simulink model "wiper_mil"  (R2018a)
settings: Solver=FixedStepDiscrete  StartTime=0.0  StopTime=10.0  FixedStep=1  RelTol=1e-3
undefined symbols (not defined in the file): sigbuilder_block
settings Model: Creator=Admin  LastModifiedBy=Admin
settings ConfigComp: CovEnable=on  RecordCoverage=on  CovMetricSettings=dcmwe  CovModelRefEnable=on

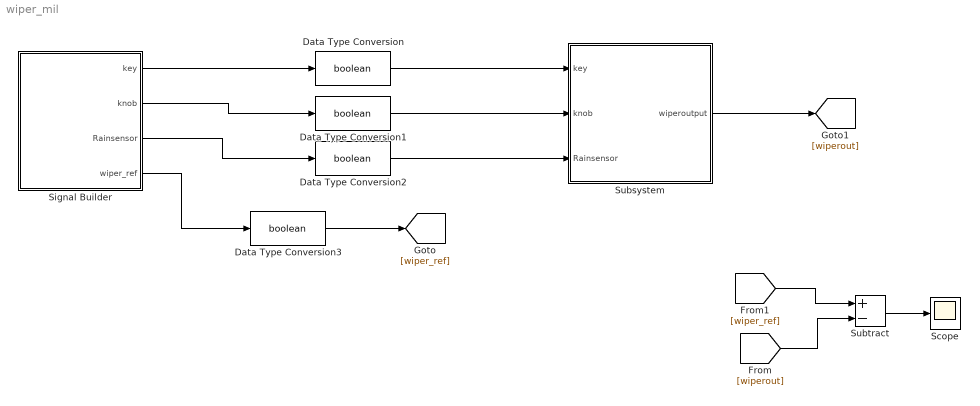
== system wiper_mil ==
  Data Type Conversion{,1..3} (4 alike) : DataTypeConversion  OutDataTypeStr=boolean
  Scope : Scope
  Signal Builder : Subsystem  Tag=STV Subsys  LoadFcn=sigbuilder_block('load',[440.25 156.75 544.5 355.5 ]);  StartFcn=sigbuilder_block('start');  StopFcn=sigbuilder_block('stop');  ClipboardFcn=sigbuilder_block('clipboard');  mask(Sigbuilder block){tuvar=[0:10]}
      mask help: Simulink:masks:SigbuilderBlock_MD
      mask init:
      | if ~strcmp(get_param(bdroot(gcbh),'SimulationStatus'),'stopped') tuvar = sigbuilder_block('maskInit'); end
      settings: CopyFcn=sigbuilder_block('copy');  DeleteFcn=sigbuilder_block('delete');  ModelCloseFcn=sigbuilder_block('modelClose');  PreSaveFcn=sigbuilder_block('preSave');  PauseFcn=sigbuilder_block('pause');  ContinueFcn=sigbuilder_block('continue');  NameChangeFcn=sigbuilder_block('namechange');  OpenFcn=sigbuilder_block('open',[440.25 156.75 544.5 355.5 ]);  CloseFcn=sigbuilder_block('close');
      mask Display: plot(0, 0, 100, 100,[2, 2, 32, 32, 2], [68, 8, 8, 68, 68],[32, 2], [38, 38], [32, 19, 2],[53, 60, 44], [32, 17, 17, 2],[16, 16, 31, 31]);txt = getActiveGroup(gcbh);text(2, 100, txt,'verticalAlignment', 'top');
  Subsystem : Subsystem
  Subtract : Sum  Inputs=+-
  wires:
  Signal Builder/1(key) -> Data Type Conversion/1
  Signal Builder/2(knob) -> Data Type Conversion1/1
  Signal Builder/3(Rainsensor) -> Data Type Conversion2/1
  Signal Builder/4(wiper_ref) -> Data Type Conversion3/1
  Data Type Conversion3/1 -> [wiper_ref]
  Data Type Conversion/1 -> Subsystem/1(key)
  Data Type Conversion1/1 -> Subsystem/2(knob)
  Data Type Conversion2/1 -> Subsystem/3(Rainsensor)
  Subsystem/1(wiperoutput) -> [wiperout]
  [wiper_ref] -> Subtract/1
  [wiperout] -> Subtract/2
  Subtract/1 -> Scope/1

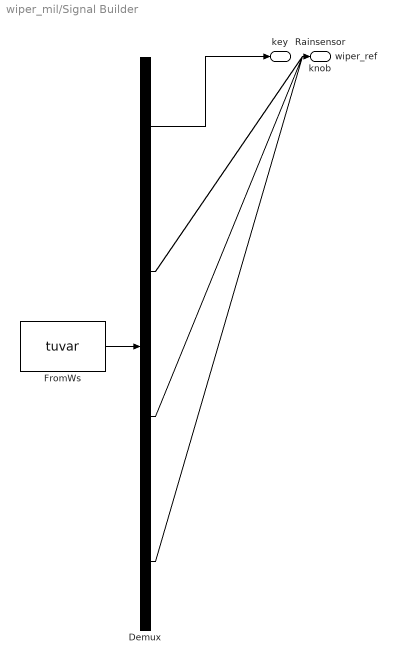
== system wiper_mil/Signal Builder ==
  Demux : Demux  Tag=STV Demux
  FromWs : FromWorkspace  Tag=STV FromWs  VariableName=tuvar  SampleTime=0
      SigBuilderData=|
      | common.afterFinalStr = 'Extrapolate'
      | common.sampleTime = 0
      | dataSet.timeRange = [0 7]
      | dataSet.name = 'Sheet1'
      | sbobj.Name = 'Signal Builder'
      | sbobj.Groups.Name = 'Sheet1'
      | sbobj.Groups.Signals(1).Name = 'key'
      | sbobj.Groups.Signals(1).XData = [0 1 2 3 4 5 6 7]
      | sbobj.Groups.Signals(1).YData = [1 1 1 1 0 0 0 0]
      | sbobj.Groups.Signals(2).Name = 'knob'
      | sbobj.Groups.Signals(2).XData = [0 1 2 3 4 5 6 7]
      | sbobj.Groups.Signals(2).YData = [1 1 0 0 1 1 0 0]
      | sbobj.Groups.Signals(3).Name = 'Rainsensor'
      | sbobj.Groups.Signals(3).XData = [0 1 2 3 4 5 6 7]
      | sbobj.Groups.Signals(3).YData = [1 0 1 0 0 1 1 0]
      | sbobj.Groups.Signals(4).Name = 'wiper_ref'
      | sbobj.Groups.Signals(4).XData = [0 1 2 3 4 5 6 7]
      | sbobj.Groups.Signals(4).YData = [1 1 1 0 0 0 0 0]
      | sbobj.Groups.TimeRange = [0 7]
  key : Outport  Tag=STV Outport
  knob : Outport  Tag=STV Outport  Port=2
  Rainsensor : Outport  Tag=STV Outport  Port=3
  wiper_ref : Outport  Tag=STV Outport  Port=4
  wires:
  Demux/1 -> key/1
  FromWs/1 -> Demux/1
  Demux/2 -> knob/1
  Demux/3 -> Rainsensor/1
  Demux/4 -> wiper_ref/1

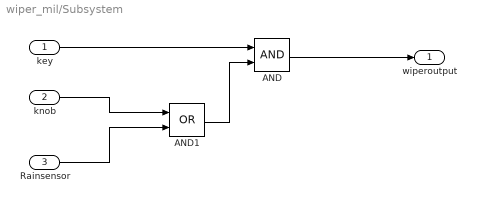
== system wiper_mil/Subsystem ==
  key : Inport
  knob : Inport  Port=2
  Rainsensor : Inport  Port=3
  AND : Logic  AllPortsSameDT=off  OutDataTypeStr=boolean
  AND1 : Logic  Operator=OR  AllPortsSameDT=off  OutDataTypeStr=boolean
  wiperoutput : Outport
  wires:
  knob/1 -> AND1/1
  key/1 -> AND/1
  AND/1 -> wiperoutput/1
  AND1/1 -> AND/2
  Rainsensor/1 -> AND1/2
